simulink library "linear_att_ctl_lib"  (R2015b)
settings: Solver=VariableStepAuto  StartTime=0.0  StopTime=10.0  RelTol=1e-3
undefined symbols (not defined in the file): tun_ctl_att_Ti, tun_ctl_att_Tp, tun_ctl_omega_kd, tun_ffp_veh_inertia_matrix_inv
settings Model: Creator=jfusco1  LastModifiedBy=jfusco1

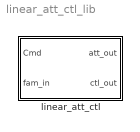
== system linear_att_ctl_lib ==
  linear_att_ctl : Subsystem

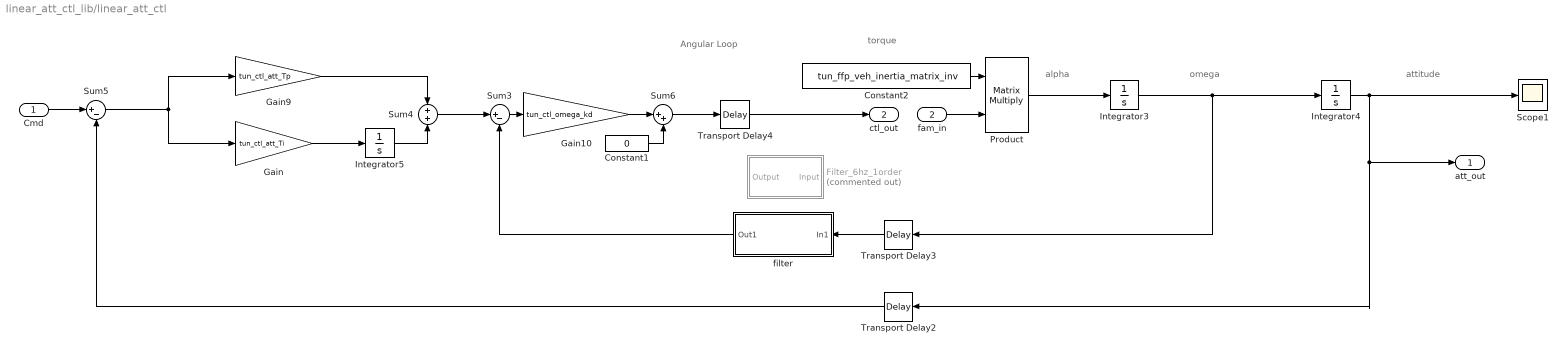
== system linear_att_ctl_lib/linear_att_ctl ==
  note: torque
  note: alpha
  note: omega
  note: attitude
  note: Angular Loop
  Cmd : Inport
  fam_in : Inport  Port=2  PortDimensions=3
  Constant1 : Constant  Value=0
  Constant2 : Constant  Value=tun_ffp_veh_inertia_matrix_inv
  Filter_6hz_1order : Subsystem  Tag=FilterWizardSubSystem  Commented=on
      settings: ErrorFcn=dspFilterRealizedInBasicElemsAlgLoopErrFcnCallback
  Gain : Gain  Gain=tun_ctl_att_Ti
  Gain10 : Gain  Gain=tun_ctl_omega_kd
  Gain9 : Gain  Gain=tun_ctl_att_Tp
  Integrator3 : Integrator
  Integrator4 : Integrator
  Integrator5 : Integrator
  Product : Product  Multiplication=Matrix(*)
  Scope1 : Scope
  Sum3 : Sum  Inputs=|+-
  Sum4 : Sum  Inputs=+|+
  Sum5 : Sum  Inputs=|+-
  Sum6 : Sum  Inputs=|++
  Transport Delay2 : TransportDelay  DelayTime=1/62.5  PadeOrder=5
  Transport Delay3 : TransportDelay  DelayTime=1/62.5  PadeOrder=5
  Transport Delay4 : TransportDelay  DelayTime=1/62.5  PadeOrder=5
  filter : Subsystem  TreatAsAtomicUnit=on
  att_out : Outport
  ctl_out : Outport  Port=2
  wires:
  Sum4/1 -> Sum3/1
  Sum5/1 -> Gain/1, Gain9/1
  Integrator4/1 -> att_out/1, Transport Delay2/1, Scope1/1
  Transport Delay4/1 -> ctl_out/1
  Product/1 -> Integrator3/1
  Gain/1 -> Integrator5/1
  Integrator5/1 -> Sum4/2
  Gain9/1 -> Sum4/1
  Gain10/1 -> Sum6/1
  Sum6/1 -> Transport Delay4/1
  Constant1/1 -> Sum6/2
  Cmd/1 -> Sum5/1
  fam_in/1 -> Product/2
  Integrator3/1 -> Transport Delay3/1, Integrator4/1
  Constant2/1 -> Product/1
  Transport Delay2/1 -> Sum5/2
  Sum3/1 -> Gain10/1
  Transport Delay3/1 -> filter/1(In1)
  filter/1(Out1) -> Sum3/2

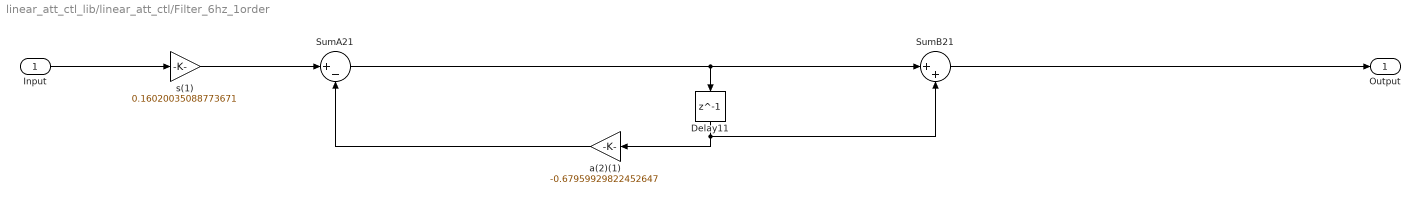
== system linear_att_ctl_lib/linear_att_ctl/Filter_6hz_1order ==
  Input : Inport
  Delay11 : Delay  DelayLength=1  InitialCondition=0
  SumA21 : Sum  Inputs=|+-  RndMeth=Nearest  SaturateOnIntegerOverflow=on  OutDataTypeStr=Inherit: Same as first input
  SumB21 : Sum  Inputs=|++  RndMeth=Nearest  SaturateOnIntegerOverflow=on  OutDataTypeStr=Inherit: Same as first input
  a(2)(1) : Gain  Gain=-0.67959929822452647  ParamDataTypeStr=double  RndMeth=Nearest  SaturateOnIntegerOverflow=on  OutDataTypeStr=Inherit: Same as input
  s(1) : Gain  Gain=0.16020035088773671  ParamDataTypeStr=double  RndMeth=Nearest  SaturateOnIntegerOverflow=on  OutDataTypeStr=Inherit: Same as input
  Output : Outport
  wires:
  Input/1 -> s(1)/1
  s(1)/1 -> SumA21/1
  SumA21/1 -> SumB21/1, Delay11/1
  SumB21/1 -> Output/1
  a(2)(1)/1 -> SumA21/2
  Delay11/1 -> a(2)(1)/1, SumB21/2

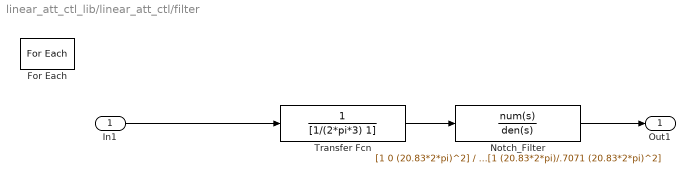
== system linear_att_ctl_lib/linear_att_ctl/filter ==
  In1 : Inport  Partition=on  PartitionDimension=1  PartitionWidth=1
  For Each : ForEach  DisableCoverage=on  IndexMode=One-based
  Notch_Filter : TransferFcn  Numerator=[1 0 (20.83*2*pi)^2]  Denominator=[1 (20.83*2*pi)/.7071 (20.83*2*pi)^2]
  Transfer Fcn : TransferFcn  Denominator=[1/(2*pi*3) 1]
  Out1 : Outport  ConcatenationDimension=1
  wires:
  Transfer Fcn/1 -> Notch_Filter/1
  In1/1 -> Transfer Fcn/1
  Notch_Filter/1 -> Out1/1
